simulink model "Control_simulation"  (R2016a)
settings: Solver=ode15s  StartTime=0.0  StopTime=40  RelTol=1e-3  AbsTol=1e-3
libraries: fl_lib x14, nesl_utility x6, pe_lib x2, elec_lib x2, simulink x2, sdl_lib x1
settings Model: Creator=matas  LastModifiedBy=matas
settings DataIOCC: LimitDataPoints=on  InspectSignalLogs=on
settings OptimizationCC: DefaultParameterBehavior=Inlined  UseDivisionForNetSlopeComputation=on  UseFloatMulNetSlope=on  InlineInvariantSignals=on  PassReuseOutputArgsAs=Individual arguments  ZeroExternalMemoryAtStartup=off  ZeroInternalMemoryAtStartup=off  NoFixptDivByZeroProtection=on  EfficientFloat2IntCast=on  OptimizeModelRefInitCode=on  LifeSpan=1
settings DebuggingCC: AllowSymbolicDim=off
settings HardwareCC: ProdBitPerPointer=32  ProdLargestAtomicInteger=Long  ProdLargestAtomicFloat=Double  ProdWordSize=32  ProdHWDeviceType=ARM Compatible->ARM Cortex
settings RTWCC: SystemTargetFile=ert.tlc  TemplateMakefile=ert_default_tmf  GenerateReport=on  IncludeHyperlinkInReport=on  LaunchReport=on  GenerateTraceInfo=on  GenerateTraceReport=on  GenerateTraceReportSl=on  GenerateTraceReportSf=on  GenerateTraceReportEml=on  GenerateCodeMetricsReport=on
settings CodeAppCC: ForceParamTrailComments=on  IgnoreCustomStorageClasses=off  OperatorAnnotations=on  SimulinkDataObjDesc=on  SFDataObjDesc=on  MATLABFcnDesc=on  CustomSymbolStrGlobalVar=rt$N$M  CustomSymbolStrType=$N$M  CustomSymbolStrFcn=$N$M$F  CustomSymbolStrMacro=$N$M  InsertBlockDesc=on  MATLABSourceComments=on
settings ERTTargetCC: GenerateSampleERTMain=on  IncludeMdlTerminateFcn=off  CombineSignalStateStructs=on  SupportAbsoluteTime=off  SupportComplex=off  SupportContinuousTime=on  InlinedParameterPlacement=NonHierarchical  ERTCustomFileTemplate=example_file_process.tlc  ERTFilePackagingFormat=CompactWithDataFile
settings ConfigComp: CovModelRefEnable=Off  CovSFcnEnable=off
settings SimscapeCC: SimscapeLogType=all  SimscapeLogDataHistory=10000

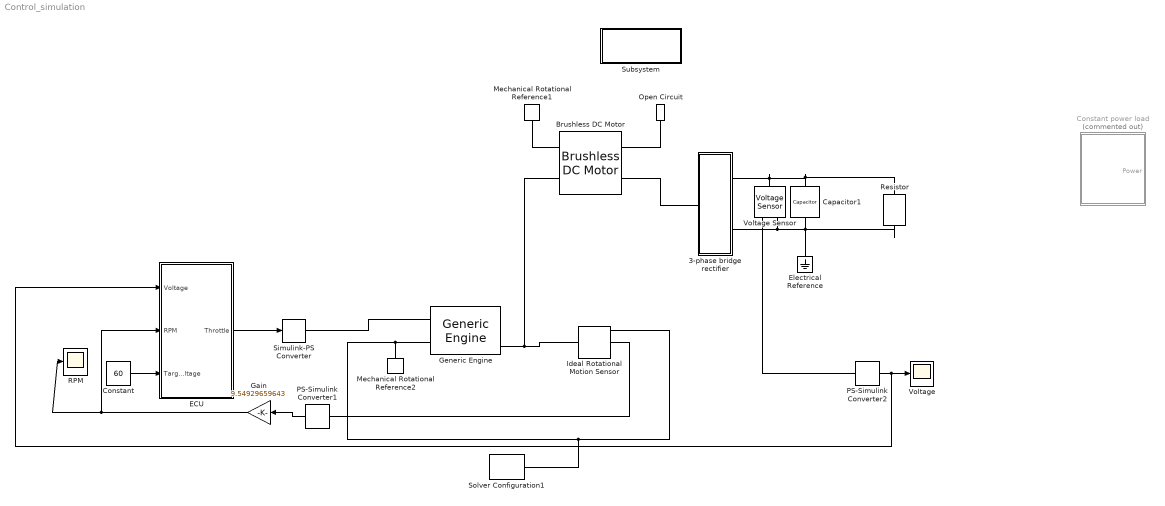
== system Control_simulation ==
  3-phase bridge rectifier : Subsystem
  Brushless DC Motor : pe_lib/Machines/Permanent Magnet Rotor/Brushless DC Motor  rotor_param=2  pm_flux_linkage=0.03 Wb  theta_constant=pi / 12 rad  emf_max=4.44 V  DphiDtheta_tab=[0.0, -0.1528, -0.1528, 0.1528, 0.1528, 0.0] Wb/rad  back_emf_tab=[0.0, 9.6, 9.6, -9.6, -9.6, 0.0] V  rotor_angle_tab=[0.0, 7.5, 22.5, 37.5, 52.5, 60.0] deg  w_meas=600 rpm  nPolePairs=6  stator_param=1  Ld=0.00022 H  Lq=0.00022 H  L0=0.00016 H  Ls=0.0002 H  Lm=0 H  Ms=0.00002 H  Rs=0.137 Ohm  initial_currents=[0.0, 0.0, 0.0] A  axes_param=2  angular_position0=0 deg
  Capacitor1 : elec_lib/Passive Devices/Capacitor  enable_table=0  c=1000 uF  Cvec=[ 1e-5 1e-6 ] F  Vvec=[ 0 10 ] V  CV_table_symmetry=1  C_tol=5  enable_C_tol=0  tol_distribution=1  nSigma=4  r=1e-6 Ohm  g=0 1/Ohm  initV=0 V  enable_operating_limits=0  operating_limit_action=2  max_working_voltage_range=[ -25 25 ] V  power_rating=1 W  enable_faults=0  fault_action=1  Cscale_faulted=100  R_faulted=0.001 Ohm  G_faulted=0 1/Ohm  tau_fault=0.001 s  enable_temporal_fault=0  t_fault=1 s  enable_behavioral_fault=0  max_permissible_voltage_range=[ -100 100 ] V  t_fail_on_voltage=1 s
  Constant : Constant  Value=60
  Constant power load : Subsystem  Commented=on
  ECU : Subsystem
  Electrical Reference : fl_lib/Electrical/Electrical Elements/Electrical Reference
  Gain : Gain  Gain=9.54929659643
  Generic Engine : sdl_lib/Engines/Generic Engine  model_parameterization=1  engine_type=1  P_max=2000 W  w_P_max=9000 rpm  w_max=9500 rpm  w_min=500 rpm  w_tab=[ 500 1000 2e+3 3e+3 4e+3 5e+3 6e+3 7e+3 ] rpm  trq_tab=[ 380 380 380 380 350 280 200 80 ] N*m  pwr_tab=[ 2e+4 4e+4 7.8e+4 1.2e+5 1.45e+5 1.48e+5 1.25e+5 6e+4 ] W  interp_method=1  model_inertia=1  inertia=0.02 kg*m^2  initial_velocity=3000 rpm  model_time_constant=1  time_constant=0.2 s  T0=0  w_thr=100 rpm  idle_speed=0  idle_speed_reference=1000 rpm  tau_controller=1 s  idle_w_thr=1 rpm  fc_model=1  fc_per_rev=25 mg/rev  displaced_volume=400 cm^3  rev_per_cycle=2  fc_w_tab=[ 1000 2e+3 3e+3 4e+3 5e+3 6e+3 ] rpm  fc_trq_tab=[ 0 80 160 200 240 320 360 400 ] N*m  fc_tab=[ 0.5 0.9 1.4 1.6 1.9 2.7 3.4 4.4; 1 1.7 2.7 3.1 3.6 5 6 7.4; 1.4 2.7 4 4.8 5.6 7.5 8.5 10.5; 2 3.6 5.8 6.7 8 10.4 11.7 13.3; 2.5 4.8 7.9 9.4 10.8 14 16.2 18.6; 3.1 6 10.3 11.9 13.8 18.4 22 26.5 ] g/s  bmep_tab=[ 0 250 500 625 750 1000 1.15e+3 1.25e+3 ] kPa  bsfc_tab=[ 410 380 300 280 270 290 320 380; 410 370 290 270 260 270 285 320; 415 380 290 275 265 270 270 300; 420 390 310 290 285 280 280 285; 430 410 340 320 310 300 310 320; 450 430 370 340 330 330 350 380 ] g/hr/kW  fc_interp_method=1
  Ideal Rotational Motion Sensor : fl_lib/Mechanical/Mechanical Sensors/Ideal Rotational Motion Sensor  offset=0 rad
  Mechanical Rotational Reference1 : fl_lib/Mechanical/Rotational Elements/Mechanical Rotational Reference
  Mechanical Rotational Reference2 : fl_lib/Mechanical/Rotational Elements/Mechanical Rotational Reference
  Open Circuit : fl_lib/Electrical/Electrical Elements/Open Circuit  v_specify=off  v_priority=None  v=0 V
  PS-Simulink Converter1 : nesl_utility/PS-Simulink Converter  PhysicalDomain=network_engine_domain  SubClassName=ps_output  LeftPortType=input  RightPortType=output  PseudoPeriodic=off  Frequencies=[]  Unit=1  AffineConversion=off
  PS-Simulink Converter2 : nesl_utility/PS-Simulink Converter  PhysicalDomain=network_engine_domain  SubClassName=ps_output  LeftPortType=input  RightPortType=output  PseudoPeriodic=off  Frequencies=[]  Unit=1  AffineConversion=off
  RPM : Scope
  Resistor : elec_lib/Passive Devices/Resistor  R=10 Ohm  R_tol=5  enable_R_tol=0  tol_distribution=1  nSigma=4  enable_operating_limits=0  operating_limit_action=2  max_working_voltage=100 V  power_rating=1 W  enable_faults=0  fault_action=1  R_faulted=Inf Ohm  enable_temporal_fault=0  t_fault=1 s  enable_behavioral_fault=0  max_permissible_current=1 A  t_fail_on_current=1 s  noise_mode=0  sample_time=0.001 s  repeatability=1  auto_seed=2090754141  user_seed=0  Tdevice=25 degC  alpha=0.00393 1/K  Tmeas=25 degC  thermal_mass=100 J/K  initial_temperature=25 degC  power_derating_T1=70 degC  power_derating_T2=155 degC  operating_temperature_range_vec=[ -50 150 ] degC
  Simulink-PS Converter : nesl_utility/Simulink-PS Converter  PhysicalDomain=network_engine_domain  SubClassName=ps_input  LeftPortType=input  RightPortType=output  PseudoPeriodic=off  Frequencies=[]  NoiseDistribution=none  NoiseParameters=[]  Unit=1  AffineConversion=off  InputFiltering=on  SimscapeFilterOrder=1  InputFilterTimeConstant=0.001  UdotUserProvided=1
  Solver Configuration1 : nesl_utility/Solver Configuration  PhysicalDomain=network_engine_domain  SubClassName=solver  LeftPortType=input  RightPortType=generic  Accelerate=off  Tones=[]  Harmonics=[]  SimulateNoise=off  Profile=off  UseLocalSampling=off  EnableSwitchedLinearOptims=on  FrequencyDomain=off  UseCCode=off  RelTol=0.001  AbsTol=1e-06  MinStep=1e-09  ToWorkspace=off  RevertToSquareIcSolve=off  NumHomotopyIterations=100  PhasorMode=off  PhasorModeNumHarmonics=1  OverrideAbsTol=off  DoDC=off  ResidualTolerance=1e-06  UseLocalSolver=off  LocalSolverChoice=NE_BACKWARD_EULER_ADVANCER  LocalSolverSampleTime=0.001  DoFixedCost=off  MaxNonlinIter=3  MaxModeIter=2  LinearAlgebra=Sparse  DelaysMemoryBudget=1024  AutomaticFiltering=on  FilteringTimeConstant=0.001
  Subsystem : Subsystem
      settings: OpenFcn=open_system('simscape')
      mask Display: disp(sprintf('Open Simscape\nLibrary'));
  Voltage : Scope
  Voltage Sensor : fl_lib/Electrical/Electrical Sensors/Voltage Sensor
  wires:
  PS-Simulink Converter1/1 -> Gain/1
  Gain/1 -> ECU/2(RPM), RPM/1
  PS-Simulink Converter2/1 -> ECU/1(Voltage), Voltage/1
  Constant/1 -> ECU/3(Target Voltage)
  ECU/1(Throttle) -> Simulink-PS Converter/1
  connections:
  Mechanical Rotational Reference1/LConn1 -- Brushless DC Motor/RConn2
  Brushless DC Motor/LConn1 -- 3-phase bridge rectifier/LConn1
  Brushless DC Motor/LConn2 -- Open Circuit/LConn1
  Mechanical Rotational Reference2/LConn1 -- Generic Engine/LConn2 -- Solver Configuration1/RConn1 -- Ideal Rotational Motion Sensor/RConn1
  Generic Engine/RConn3 -- Brushless DC Motor/RConn1 -- Ideal Rotational Motion Sensor/LConn1
  Ideal Rotational Motion Sensor/RConn2 -- PS-Simulink Converter1/LConn1
  Capacitor1/LConn1 -- Resistor/LConn1 -- Voltage Sensor/LConn1 -- 3-phase bridge rectifier/RConn1
  3-phase bridge rectifier/RConn2 -- Voltage Sensor/RConn2 -- Resistor/RConn1 -- Electrical Reference/LConn1 -- Capacitor1/RConn1
  Voltage Sensor/RConn1 -- PS-Simulink Converter2/LConn1
  Simulink-PS Converter/RConn1 -- Generic Engine/LConn1

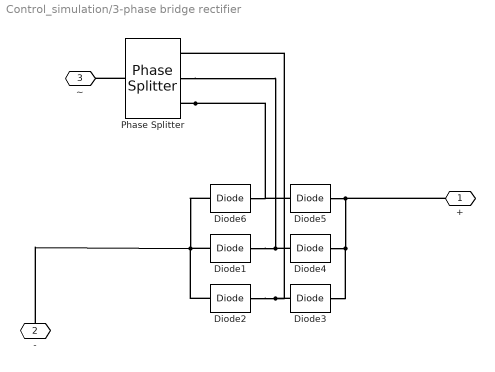
== system Control_simulation/3-phase bridge rectifier ==
  Diode{1..6} (6 alike) : fl_lib/Electrical/Electrical Elements/Diode  Vf=0.6 V  Ron=0.3 Ohm  Goff=1e-8 1/Ohm  i_specify=off  i_priority=None  i=0 A  v_specify=off  v_priority=None  v=0 V
  Phase Splitter : pe_lib/Connections/Phase Splitter
  + : PMIOPort  Port=1  Side=Right
  "- " : PMIOPort  Port=2  Side=Right
  ~ : PMIOPort  Port=3  Side=Left
  connections:
  Phase Splitter/RConn3 -- Diode5/LConn1 -- Diode6/RConn1
  "- "/RConn1 -- Diode2/LConn1 -- Diode1/LConn1 -- Diode6/LConn1
  Phase Splitter/RConn2 -- Diode4/LConn1 -- Diode1/RConn1
  Diode2/RConn1 -- Phase Splitter/RConn1 -- Diode3/LConn1
  +/RConn1 -- Diode5/RConn1 -- Diode4/RConn1 -- Diode3/RConn1
  Phase Splitter/LConn1 -- ~/RConn1

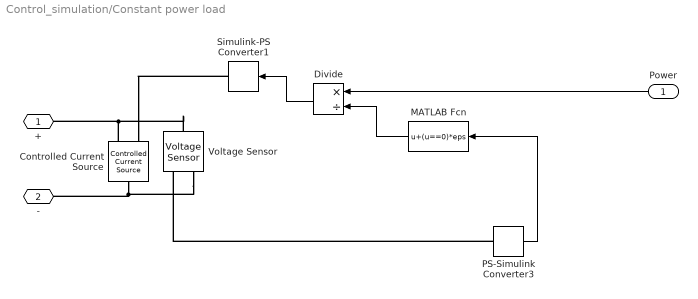
== system Control_simulation/Constant power load ==
  Power : Inport
  Controlled Current Source : fl_lib/Electrical/Electrical Sources/Controlled Current Source
  Divide : Product  Inputs=*/
  MATLAB Fcn : MATLABFcn  MATLABFcn=u+(u==0)*eps
  PS-Simulink Converter3 : nesl_utility/PS-Simulink Converter  PhysicalDomain=network_engine_domain  SubClassName=ps_output  LeftPortType=input  RightPortType=output  PseudoPeriodic=off  Frequencies=[]  Unit=1  AffineConversion=off
  Simulink-PS Converter1 : nesl_utility/Simulink-PS Converter  PhysicalDomain=network_engine_domain  SubClassName=ps_input  LeftPortType=input  RightPortType=output  PseudoPeriodic=off  Frequencies=[]  NoiseDistribution=none  NoiseParameters=[]  Unit=1  AffineConversion=off  InputFiltering=off  SimscapeFilterOrder=1  InputFilterTimeConstant=0.001  UdotUserProvided=1
  Voltage Sensor : fl_lib/Electrical/Electrical Sensors/Voltage Sensor
  + : PMIOPort  Port=1  Side=Right
  - : PMIOPort  Port=2  Side=Right
  wires:
  Divide/1 -> Simulink-PS Converter1/1
  MATLAB Fcn/1 -> Divide/2
  PS-Simulink Converter3/1 -> MATLAB Fcn/1
  Power/1 -> Divide/1
  connections:
  Voltage Sensor/RConn2 -- -/RConn1 -- Controlled Current Source/LConn1
  Voltage Sensor/LConn1 -- +/RConn1 -- Controlled Current Source/RConn2
  PS-Simulink Converter3/LConn1 -- Voltage Sensor/RConn1
  Simulink-PS Converter1/RConn1 -- Controlled Current Source/RConn1

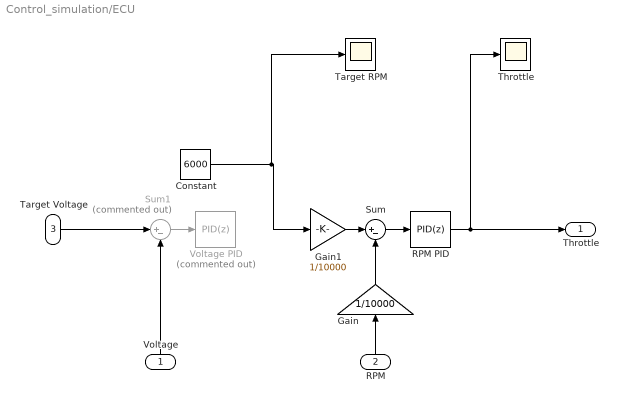
== system Control_simulation/ECU ==
  Voltage : Inport
  RPM : Inport  Port=2
  Target Voltage : Inport  Port=3
  Constant : Constant  Value=6000
  Gain : Gain  Gain=1/10000
  Gain1 : Gain  Gain=1/10000
  RPM PID : simulink/Continuous/PID Controller  Controller=PID  TimeDomain=Discrete-time  SampleTime=0.02  IntegratorMethod=Forward Euler  FilterMethod=Forward Euler  Form=Parallel  UseFilter=off  ControllerParametersSource=internal  P=0.02  I=0.00604552334869684  D=0.00326053181479634  N=4221.52793378059  InitialConditionSource=internal  InitialConditionForIntegrator=0  InitialConditionForFilter=0  ExternalReset=none  ZeroCross=off  LimitOutput=on  UpperSaturationLimit=1  LowerSaturationLimit=0  LinearizeAsGain=on  AntiWindupMode=clamping  Kb=1  TrackingMode=off  Kt=1  PParamMin=[]  PParamMax=[]  IParamMin=[]  IParamMax=[]  DParamMin=[]  DParamMax=[]  NParamMin=[]  NParamMax=[]  KbParamMin=[]  KbParamMax=[]  KtParamMin=[]  KtParamMax=[]  POutMin=[]  POutMax=[]  IOutMin=[]  IOutMax=[]  DOutMin=[]  DOutMax=[]  NOutMin=[]  NOutMax=[]  KbOutMin=[]  KbOutMax=[]  KtOutMin=[]  KtOutMax=[]  IntegratorOutMin=[]  IntegratorOutMax=[]  FilterOutMin=[]  FilterOutMax=[]  SumOutMin=[]  SumOutMax=[]  SumI1OutMin=[]  SumI1OutMax=[]  SumI2OutMin=[]  SumI2OutMax=[]  SumI3OutMin=[]  SumI3OutMax=[]  SumDOutMin=[]  SumDOutMax=[]  SaturationOutMin=[]  SaturationOutMax=[]  IntegratorContinuousStateAttributes=''  IntegratorStateMustResolveToSignalObject=off  IntegratorRTWStateStorageClass=Auto  FilterContinuousStateAttributes=''  FilterStateMustResolveToSignalObject=off  FilterRTWStateStorageClass=Auto  DifferentiatorICPrevScaledInput=0  DifferentiatorOutMin=[]  DifferentiatorOutMax=[]
  Sum : Sum  Inputs=|+-
  Sum1 : Sum  Commented=on  Inputs=|+-
  Target RPM : Scope
  "Throttle " : Scope
  Voltage PID : simulink/Continuous/PID Controller  Commented=on  Controller=PID  TimeDomain=Discrete-time  SampleTime=0.02  IntegratorMethod=Forward Euler  FilterMethod=Forward Euler  Form=Parallel  UseFilter=off  ControllerParametersSource=internal  P=100  I=100  D=0  N=100  InitialConditionSource=internal  InitialConditionForIntegrator=0  InitialConditionForFilter=0  ExternalReset=none  LimitOutput=on  UpperSaturationLimit=9000  LowerSaturationLimit=2000  LinearizeAsGain=on  AntiWindupMode=clamping  Kb=1  TrackingMode=off  Kt=1  PParamMin=[]  PParamMax=[]  IParamMin=[]  IParamMax=[]  DParamMin=[]  DParamMax=[]  NParamMin=[]  NParamMax=[]  KbParamMin=[]  KbParamMax=[]  KtParamMin=[]  KtParamMax=[]  POutMin=[]  POutMax=[]  IOutMin=[]  IOutMax=[]  DOutMin=[]  DOutMax=[]  NOutMin=[]  NOutMax=[]  KbOutMin=[]  KbOutMax=[]  KtOutMin=[]  KtOutMax=[]  IntegratorOutMin=[]  IntegratorOutMax=[]  FilterOutMin=[]  FilterOutMax=[]  SumOutMin=[]  SumOutMax=[]  SumI1OutMin=[]  SumI1OutMax=[]  SumI2OutMin=[]  SumI2OutMax=[]  SumI3OutMin=[]  SumI3OutMax=[]  SumDOutMin=[]  SumDOutMax=[]  SaturationOutMin=[]  SaturationOutMax=[]  IntegratorContinuousStateAttributes=''  IntegratorStateMustResolveToSignalObject=off  IntegratorRTWStateStorageClass=Auto  FilterContinuousStateAttributes=''  FilterStateMustResolveToSignalObject=off  FilterRTWStateStorageClass=Auto  DifferentiatorICPrevScaledInput=0  DifferentiatorOutMin=[]  DifferentiatorOutMax=[]
  Throttle : Outport
  wires:
  RPM PID/1 -> Throttle/1, "Throttle "/1
  Target Voltage/1 -> Sum1/1
  Sum1/1 -> Voltage PID/1
  Sum/1 -> RPM PID/1
  Voltage/1 -> Sum1/2
  RPM/1 -> Gain/1
  Gain/1 -> Sum/2
  Gain1/1 -> Sum/1
  Constant/1 -> Target RPM/1, Gain1/1

== system Control_simulation/Subsystem ==
